simulink model "yang_ref2"  (Simulink 3.00)
settings: Solver=ode45  StartTime=0.0  StopTime=10.0  RelTol=1e-3
settings Model: LastModifiedBy=Administrator

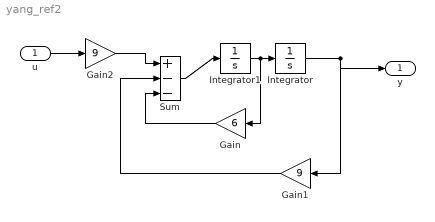
== system yang_ref2 ==
  u : Inport  Port=1  PortWidth=-1  SampleTime=-1  DataType=auto
      settings: SignalType=auto
  Gain : Gain  Orientation=left  Gain=6  SaturateOnIntegerOverflow=on
  Gain1 : Gain  Orientation=left  Gain=9  SaturateOnIntegerOverflow=on
  Gain2 : Gain  Gain=9  SaturateOnIntegerOverflow=on
  Integrator : Integrator  ExternalReset=none  InitialConditionSource=internal  InitialCondition=0  LimitOutput=off  UpperSaturationLimit=inf  LowerSaturationLimit=-inf  ShowSaturationPort=off  ShowStatePort=off  AbsoluteTolerance=auto
  Integrator1 : Integrator  ExternalReset=none  InitialConditionSource=internal  InitialCondition=0  LimitOutput=off  UpperSaturationLimit=inf  LowerSaturationLimit=-inf  ShowSaturationPort=off  ShowStatePort=off  AbsoluteTolerance=auto
  Sum : Sum  Inputs=+--  SaturateOnIntegerOverflow=on
  y : Outport  Port=1
  wires:
  Integrator/1 -> y/1, Gain1/1
  Sum/1 -> Integrator1/1
  Gain1/1 -> Sum/2
  Integrator1/1 -> Integrator/1, Gain/1
  Gain/1 -> Sum/3
  Gain2/1 -> Sum/1
  u/1 -> Gain2/1
